simulink model "c_citation"  (R2020a)
settings: Solver=ode5  StartTime=0.0  StopTime=inf  FixedStep=0.01  RelTol=1e-3
InitFcn:
  | load('simulation_parameters');
values from neighbouring files (symbols this model uses):
  chord = 1.991    [citdata.mat]
  cv1 = 20000    [gear_params.m]
  cv2 = cv1    (= 20000)    [gear_params.m]
  cv3 = 4000    [gear_params.m]
  cv4 = 20000    [gear_params.m]
  deltagmax1 = 0.25    [gear_params.m]
  deltagmax2 = deltagmax1    (= 0.25)    [gear_params.m]
  deltagmax3 = 0.24    [gear_params.m]
  deltagmax4 = 0.02    [gear_params.m]
  ealphag = [0  0.2618  0.6981; 1  1.3  0.8]    [citdata.mat]
  ealphas = [0  0.2618  0.6981; 0.157  0.157  0.175]    [citdata.mat]
  g0 = 9.80665    [ac_genrl.mat]
  hDME = 0    [ac_genrl.mat]
  hGS = 0    [ac_genrl.mat]
  kt1 = 525020    [gear_params.m]
  kt2 = kt1    (= 525020)    [gear_params.m]
  kt3 = 457050    [gear_params.m]
  lh = 5.53    [citdata.mat]
  matbuaf = [0  -0.1745  0.4363; 0  -0.1  -0.1; 0.6981  -0.1  -0.1]    [citdata.mat]
  matdaf = [0 0 0.2618 0.6981 0.734842105263 0.771584210526 0.808326315789 0.845068421053 0.881810526316 0.918552631579 0.955294736842 0.992036842105 ... (529 elements, 23x23)]    [citdata.mat]
  matdam = [0 0.05 0.15 0.25 0.35 0.45 0.55 0.65 0.75 0.803571428571 0.857142857143 0.910714285714 ... (529 elements, 23x23)]    [citdata.mat]
  matdbbf = [0 0 0.6981 0.74464 0.79118 0.83772 0.88426 0.9308 0.97734 1.02388 1.07042 1.11696 ... (324 elements, 18x18)]    [citdata.mat]
  matdeaf = [0 0 0.2618 0.6981 0.734842105263 0.771584210526 0.808326315789 0.845068421053 0.881810526316 0.918552631579 0.955294736842 0.992036842105 ... (529 elements, 23x23)]    [citdata.mat]
  matdgaf = [0 0 0.2618 0.6981 -0.1745 -0.0175 -0.008 -0.009 0.4363 -0.0175 -0.008 -0.009 ... (16 elements, 4x4)]    [citdata.mat]
  matdqaf = [0 0 0.2618 0.6981 0.734842105263 0.771584210526 0.808326315789 0.845068421053 0.881810526316 0.918552631579 0.955294736842 0.992036842105 ... (529 elements, 23x23)]    [citdata.mat]
  matduaf = [0 0 0.2618 0.6981 0.734842105263 0.771584210526 0.808326315789 0.845068421053 0.881810526316 0.918552631579 0.955294736842 0.992036842105 ... (529 elements, 23x23)]    [citdata.mat]
  matdwaw = [0 0 0.1745 0.3491 0.5236 0.6458 1.2916 -0.1745 0 0.0018 0.0046 0.0088 ... (49 elements, 7x7)]    [citdata.mat]
  matedhr = [0 1 1 0.71 2 0.51 3 0.34 5 0.12 7.5 0.03 ... (20 elements, 2x10)]    [citdata.mat]
  mateif = [0  0.2618  0.6981; 0  -0.075  -0.075]    [citdata.mat]
  matelhr = [0 1 1 0.95 2 0.91 3 0.84 5 0.71 7.5 0.35 ... (20 elements, 2x10)]    [citdata.mat]
  matemhr = [0 1 1 0.9 2 0.8 3 0.7 5 0.5 7.5 0.25 ... (20 elements, 2x10)]    [citdata.mat]
  matemv1 = [0  90  100; 0  1  1]    [citdata.mat]
  matemv2 = [20  75  90; 0  1  1]    [citdata.mat]
  matemve = [0  90  100; 0  1  1]    [citdata.mat]
  matetam = [0  -0.1745  0.4363; 0  -0.04  -0.04; 1  -0.04  -0.04]    [citdata.mat]
  mateuaf = [0 0 0.6981 0.733005 0.76791 0.802815 0.83772 0.872625 0.90753 0.942435 0.97734 1.012245 ... (529 elements, 23x23)]    [citdata.mat]
  matfaaf = [0 0 0.2618 0.6981 0.734842105263 0.771584210526 0.808326315789 0.845068421053 0.881810526316 0.918552631579 0.955294736842 0.992036842105 ... (529 elements, 23x23)]    [citdata.mat]
  matfaxl = [0.15  0.35; 1  1]    [citdata.mat]
  matibaf = [0 0 0.2618 0.6981 -0.2 -0.119 -0.117 -0.108 0.3 -0.059 -0.052 -0.038 ... (16 elements, 4x4)]    [citdata.mat]
  matibb = [0 0 0.2618 1.571 3.142 -0.2 0 0 0.074 0.124 0 0 ... (50 elements, 5x10)]    [citdata.mat]
  matibmh = [0 0 15000 17142.8571429 19285.7142857 21428.5714286 23571.4285714 25714.2857143 27857.1428571 30000 0 0 ... (100 elements, 10x10)]    [citdata.mat]
  matipaf = [0  -0.1745  0.4363; 0  -0.44  -0.44; 0.6981  -0.44  -0.44]    [citdata.mat]
  matipmh = [0 0 15000 17142.8571429 19285.7142857 21428.5714286 23571.4285714 25714.2857143 27857.1428571 30000 0 0 ... (100 elements, 10x10)]    [citdata.mat]
  matiraf = [0 0 0.2618 0.6981 -0.2 0.05 -0.03 0.01 0.3 0.3 0.37 0.41 ... (16 elements, 4x4)]    [citdata.mat]
  matiuaf = [0  -0.2  0.3; 0  0.052  -0.003; 0.6981  0.052  -0.003]    [citdata.mat]
  matiwaf = [0  -0.1745  0.4363; 0  -0.185  -0.185; 0.6981  -0.185  -0.185]    [citdata.mat]
  matlaf = [0 0 0.2618 0.6981 0.734842105263 0.771584210526 0.808326315789 0.845068421053 0.881810526316 0.918552631579 0.955294736842 0.992036842105 ... (529 elements, 23x23)]    [citdata.mat]
  matlam = [0 0.05 0.15 0.25 0.35 0.45 0.55 0.65 0.75 0.803571428571 0.857142857143 0.910714285714 ... (529 elements, 23x23)]    [citdata.mat]
  matleaf = [0 0 0.2618 0.6981 0.734842105263 0.771584210526 0.808326315789 0.845068421053 0.881810526316 0.918552631579 0.955294736842 0.992036842105 ... (529 elements, 23x23)]    [citdata.mat]
  matleam = [0  -0.1745  0.4363; 0  0.58  0.58; 1  0.58  0.58]    [citdata.mat]
  matlgaf = [0 0 0.2618 0.6981 -0.1745 0.045 0.105 0.14 0.4363 0.045 0.105 0.14 ... (16 elements, 4x4)]    [citdata.mat]
  matlqaf = [0 0 0.2618 0.6981 0.734842105263 0.771584210526 0.808326315789 0.845068421053 0.881810526316 0.918552631579 0.955294736842 0.992036842105 ... (529 elements, 23x23)]    [citdata.mat]
  matluaf = [0 0 0.2618 0.6981 0.734842105263 0.771584210526 0.808326315789 0.845068421053 0.881810526316 0.918552631579 0.955294736842 0.992036842105 ... (529 elements, 23x23)]    [citdata.mat]
  matmaaf = [0 0 0.2618 0.6981 0.734842105263 0.771584210526 0.808326315789 0.845068421053 0.881810526316 0.918552631579 0.955294736842 0.992036842105 ... (484 elements, 22x22)]    [citdata.mat]
  matmaam = [0 0.05 0.15 0.25 0.35 0.45 0.55 0.65 0.75 0.803571428571 0.857142857143 0.910714285714 ... (484 elements, 22x22)]    [citdata.mat]
  matmaf = [0 0 0.2618 0.6981 0.734842105263 0.771584210526 0.808326315789 0.845068421053 0.881810526316 0.918552631579 0.955294736842 0.992036842105 ... (529 elements, 23x23)]    [citdata.mat]
  matmam = [0 0.05 0.15 0.25 0.35 0.45 0.55 0.65 0.75 0.803571428571 0.857142857143 0.910714285714 ... (529 elements, 23x23)]    [citdata.mat]
  matmbbf = [0 0 0.6981 0.74464 0.79118 0.83772 0.88426 0.9308 0.97734 1.02388 1.07042 1.11696 ... (324 elements, 18x18)]    [citdata.mat]
  matmeaf = [0 0 0.2618 0.6981 0.734842105263 0.771584210526 0.808326315789 0.845068421053 0.881810526316 0.918552631579 0.955294736842 0.992036842105 ... (529 elements, 23x23)]    [citdata.mat]
  matmeam = [0 0 1 1.05 1.1 1.15 1.2 1.25 1.3 1.35 1.4 1.45 ... (529 elements, 23x23)]    [citdata.mat]
  matmgaf = [0 0 0.2618 0.6981 -0.1745 -0.01 -0.024 -0.035 0.4363 -0.01 -0.024 -0.035 ... (16 elements, 4x4)]    [citdata.mat]
  matmqaf = [0 0 0.2618 0.6981 0.734842105263 0.771584210526 0.808326315789 0.845068421053 0.881810526316 0.918552631579 0.955294736842 0.992036842105 ... (529 elements, 23x23)]    [citdata.mat]
  matmrbr = [0  0  0.5236; 0  0  0; 0.384  0.001  0.001]    [citdata.mat]
  matnbab = [0 0 0.2618 1.571 3.142 -0.2 0 0 -0.0199 -0.1049 0 0 ... (25 elements, 5x5)]    [citdata.mat]
  matnbaf = [0  -0.2  0.3; 0  0.105  0.18; 0.6981  0.105  0.18]    [citdata.mat]
  matnbmh = [0 0 15000 17142.8571429 19285.7142857 21428.5714286 23571.4285714 25714.2857143 27857.1428571 30000 0 0 ... (100 elements, 10x10)]    [citdata.mat]
  matnpaf = [0 0 0.2618 0.6981 -0.2 0.03 0.03 0.05 0.3 -0.12 -0.12 -0.2 ... (16 elements, 4x4)]    [citdata.mat]
  matnpmh = [0 0 15000 17142.8571429 19285.7142857 21428.5714286 23571.4285714 25714.2857143 27857.1428571 30000 0 0 ... (100 elements, 10x10)]    [citdata.mat]
  matnraf = [0  -0.1745  0.4363; 0  -0.21  -0.21; 0.6981  -0.21  -0.21]    [citdata.mat]
  matnuaf = [0  -0.1745  0.4363; 0  -0.101  -0.101; 0.6981  -0.101  -0.101]    [citdata.mat]
  matnwaf = [0 0 0.2618 0.6981 -0.2 -0.02 -0.037 -0.049 0.3 0.03 0.043 0.036 ... (16 elements, 4x4)]    [citdata.mat]
  matnwmh = [0 0 15000 17142.8571429 19285.7142857 21428.5714286 23571.4285714 25714.2857143 27857.1428571 30000 0 0 ... (100 elements, 10x10)]    [citdata.mat]
  matqlaf = [0  -0.1745  0.4363; 0  -1  -1; 0.6981  -1  -1]    [citdata.mat]
  matquaf = [0 0 0.6981 0.733005 0.76791 0.802815 0.83772 0.872625 0.90753 0.942435 0.97734 1.012245 ... (529 elements, 23x23)]    [citdata.mat]
  matqxl = [0.15  0.35; 1  1]    [citdata.mat]
  matqxm = [0.15  0.35; 1  1]    [citdata.mat]
  matrtam = [0  -0.1745  0.4363; 0  0.011  0.011; 1  0.011  0.011]    [citdata.mat]
  matruaf = [0  -0.1745  0.4363; 0  0.2  0.2; 0.6981  0.2  0.2]    [citdata.mat]
  matrumh = [0 0 15000 17142.8571429 19285.7142857 21428.5714286 23571.4285714 25714.2857143 27857.1428571 30000 0 0 ... (100 elements, 10x10)]    [citdata.mat]
  matuut = [0  0.5  1; 0  1.35  1]    [citdata.mat]
  matwtam = [0  -0.1745  0.4363; 0  0.011  0.011; 1  0.011  0.011]    [citdata.mat]
  matybab = [0 0 0.2618 1.571 3.142 -0.2 0 0 0.34 0.75 0 0 ... (25 elements, 5x5)]    [citdata.mat]
  matybaf = [0  -0.1745  0.4363; 0  -0.75  -0.75; 0.6981  -0.75  -0.75]    [citdata.mat]
  matyraf = [0  -0.1745  0.4363; 0  0.85  0.85; 0.6981  0.85  0.85]    [citdata.mat]
  matyuaf = [0  -0.1745  0.4363; 0  0.23  0.23; 0.6981  0.23  0.23]    [citdata.mat]
  matywaf = [0  -0.1745  0.4363; 0  -0.04  -0.04; 0.6981  -0.04  -0.04]    [citdata.mat]
  murol = 0.03*10    (= 0.3)    [gear_params.m]
  P1 = 2000    [gear_params.m]
  P2 = P1    (= 2000)    [gear_params.m]
  P3 = 2550    [gear_params.m]
  P4 = 40000    [gear_params.m]
  psiLOC = 0    [ac_genrl.mat]
  pstat0 = 101325    [ac_genrl.mat]
  S = 24.99    [citdata.mat]
  span = 13.325    [citdata.mat]
  T0 = 288.15    [ac_genrl.mat]
  tilteng = [0 0]    [citdata.mat]
  toweng = [0 0]    [citdata.mat]
  vdommyr37 = [0  0.2618  0.6981; 0  0.025  0]    [citdata.mat]
  vdommyr38 = [0  0.2618  0.6981; -0.01  0  -0.01]    [citdata.mat]
  Vw915 = 0    [initcit.m]
  winddir = 45*(pi/180)    (= 0.785398163397)    [initcit.m]
  xcgref = 6.5    [citdata.mat]
  xDME = 0    [ac_genrl.mat]
  xeng = [8.407 8.407]    [citdata.mat]
  xGS = 0    [ac_genrl.mat]
  xiacc = 3.2    [ac_genrl.mat]
  xl1 = xcg-6.858    [gear_params.m]
  xl2 = xcg-6.858    [gear_params.m]
  xl3 = xcg-2.0752    [gear_params.m]
  xl4 = xcg-12.742    [gear_params.m]
  xLOC = 0    [ac_genrl.mat]
  ycgref = 0    [citdata.mat]
  yDME = 0    [ac_genrl.mat]
  yeng = [3 -3]    [citdata.mat]
  yGS = 0    [ac_genrl.mat]
  yiacc = 0    [ac_genrl.mat]
  yl1 = 1.918    [gear_params.m]
  yl2 = -1.918    [gear_params.m]
  yl3 = 0    [gear_params.m]
  ... (+9 more)
undefined symbols (not defined in the file or in its folder): Deng, massinit, matff, matn1d, matn2d, matthr, u0, ut0, x0, xt0
(part 3 of 5)

== system c_citation/Cessna Citation 500/Citation model DASMAT/AIRCRAFT MODEL/LANDING GEAR/Landing Gear model/Left Main Gear ==
  Inputs : Inport
  Axes Transformation Heading attached vertical axis to body axis : Subsystem
  Calculation of the Moments : Subsystem
  Demux : Demux  Outputs=[6 2 5]
      settings: DisplayOption=none
  FS Side Force : Constant  Value=0
  FV Vertical Force : Subsystem
  Fmu Longitudinal Force : Fcn  Expr=u[1]*murol
  Mux : Mux  Inputs=3
  Mux1 : Mux  Inputs=2
  Terminator : Terminator
  Terminator1 : Terminator
  FX FY FZ : Outport  VectorParamsAs1DForOutWhenUnconnected=off
  L M N : Outport  Port=2  VectorParamsAs1DForOutWhenUnconnected=off
  wires:
  Fmu Longitudinal Force/1 -> Mux/1
  FS Side Force/1 -> Mux/2
  FV Vertical Force/1(Out1) -> Fmu Longitudinal Force/1, Mux/3
  Calculation of the Moments/1(L M N) -> L M N/1
  Inputs/1 -> FV Vertical Force/1(In1), Demux/1
  Demux/1 -> Terminator/1
  Demux/3 -> Terminator1/1
  Mux1/1 -> Axes Transformation Heading attached vertical axis to body axis/1(Fmu FS FV phi theta)
  Mux/1 -> Mux1/1
  Demux/2 -> Mux1/2  "phi theta"
  Axes Transformation Heading attached vertical axis to body axis/1(FX FY FZ) -> FX FY FZ/1, Calculation of the Moments/1(FX FY FZ)

== system c_citation/Cessna Citation 500/Citation model DASMAT/AIRCRAFT MODEL/LANDING GEAR/Landing Gear model/Nose Gear ==
  Inputs : Inport
  Axes Transformation Heading attached vertical axis to body axis : Subsystem
  Calculation of the Moments : Subsystem
  Demux : Demux  Outputs=[6 2 5]
      settings: DisplayOption=none
  F Vertical Force : Subsystem
  FS Side Force : Constant  Value=0
  Fmu Longitudinal Force : Fcn  Expr=u[1]*murol
  Mux : Mux  Inputs=3
  Mux1 : Mux  Inputs=2
  Terminator : Terminator
  Terminator1 : Terminator
  FX FY FZ : Outport  VectorParamsAs1DForOutWhenUnconnected=off
  L M N : Outport  Port=2  VectorParamsAs1DForOutWhenUnconnected=off
  wires:
  Fmu Longitudinal Force/1 -> Mux/1
  FS Side Force/1 -> Mux/2
  F Vertical Force/1(Out1) -> Fmu Longitudinal Force/1, Mux/3
  Calculation of the Moments/1(L M N) -> L M N/1
  Inputs/1 -> F Vertical Force/1(In1), Demux/1
  Demux/1 -> Terminator/1
  Demux/3 -> Terminator1/1
  Mux1/1 -> Axes Transformation Heading attached vertical axis to body axis/1(Fmu FS FV phi theta)
  Mux/1 -> Mux1/1
  Demux/2 -> Mux1/2  "phi theta"
  Axes Transformation Heading attached vertical axis to body axis/1(FX FY FZ) -> FX FY FZ/1, Calculation of the Moments/1(FX FY FZ)

== system c_citation/Cessna Citation 500/Citation model DASMAT/AIRCRAFT MODEL/LANDING GEAR/Landing Gear model/Right Main Gear ==
  Inputs : Inport
  Axes Transformation Heading attached vertical axis to body axis : Subsystem
  Calculation of the Moments : Subsystem
  Demux : Demux  Outputs=[6 2 5]
      settings: DisplayOption=none
  FS Side Force : Constant  Value=0
  FV Vertical Force : Subsystem
  Fmu Longitudinal Force : Fcn  Expr=u[1]*murol
  Mux : Mux  Inputs=3
  Mux1 : Mux  Inputs=2
  Terminator : Terminator
  Terminator1 : Terminator
  FX FY FZ : Outport  VectorParamsAs1DForOutWhenUnconnected=off
  L M N : Outport  Port=2  VectorParamsAs1DForOutWhenUnconnected=off
  wires:
  Fmu Longitudinal Force/1 -> Mux/1
  FS Side Force/1 -> Mux/2
  FV Vertical Force/1(Out1) -> Fmu Longitudinal Force/1, Mux/3
  Calculation of the Moments/1(L M N) -> L M N/1
  Inputs/1 -> FV Vertical Force/1(In1), Demux/1
  Demux/1 -> Terminator/1
  Demux/3 -> Terminator1/1
  Mux1/1 -> Axes Transformation Heading attached vertical axis to body axis/1(Fmu FS FV phi theta)
  Mux/1 -> Mux1/1
  Demux/2 -> Mux1/2  "phi theta"
  Axes Transformation Heading attached vertical axis to body axis/1(FX FY FZ) -> FX FY FZ/1, Calculation of the Moments/1(FX FY FZ)

== system c_citation/Cessna Citation 500/Citation model DASMAT/AIRCRAFT MODEL/LANDING GEAR/Landing Gear model/Tail Scraper ==
  Inputs : Inport
  Axes Transformation Heading attached vertical axis to body axis : Subsystem
  Calculation of the Moments : Subsystem
  Demux : Demux  Outputs=[6 2 5]
      settings: DisplayOption=none
  FS Side Force : Constant  Value=0
  FV Vertical Force : Subsystem
  Fmu : Constant  Value=0
  Mux : Mux  Inputs=3
  Mux1 : Mux  Inputs=2
  Terminator : Terminator
  Terminator1 : Terminator
  FX FY FZ : Outport  VectorParamsAs1DForOutWhenUnconnected=off
  L M N : Outport  Port=2  VectorParamsAs1DForOutWhenUnconnected=off
  wires:
  Fmu/1 -> Mux/1
  FS Side Force/1 -> Mux/2
  Calculation of the Moments/1(L M N) -> L M N/1
  Inputs/1 -> FV Vertical Force/1(In1), Demux/1
  Demux/1 -> Terminator/1
  Demux/3 -> Terminator1/1
  Mux1/1 -> Axes Transformation Heading attached vertical axis to body axis/1(Fmu FS FV phi theta)
  Mux/1 -> Mux1/1
  Demux/2 -> Mux1/2  "phi theta"
  Axes Transformation Heading attached vertical axis to body axis/1(FX FY FZ) -> FX FY FZ/1, Calculation of the Moments/1(FX FY FZ)
  FV Vertical Force/1(Out1) -> Mux/3

== system c_citation/Cessna Citation 500/Citation model DASMAT/AIRCRAFT MODEL/WIND//TURBULENCE/Logarithmic Wind model/Logarithmic Wind model ==
  note: winddir output deleted
      | you can calculate it yourself
      | from uvw, you lazy bastard
  note: runway elevation
      | correction deleted,
      | is all relative to sea level
  he : Inport
  Constant : Constant  Value=0
  Mux : Mux  Inputs=2
  Product : Product  InputSameDT=on  SaturateOnIntegerOverflow=on  OutDataTypeStr=Inherit: Same as first input
  Switch : Switch  Threshold=300  SaturateOnIntegerOverflow=on  InputSameDT=on
  Vwind above 300m : Fcn  Expr=1.637
  Vwind below 300m : Fcn  Expr=(0.43*log10(u)+0.572)
  Vwind915 : Subsystem
  Windddirection : Subsystem
  uwind earth axis : Fcn  Expr=cos(u[1])*u[2]
  vwind earth axis : Fcn  Expr=sin(u[1])*u[2]
  uwind : Outport  VectorParamsAs1DForOutWhenUnconnected=off
  vwind : Outport  Port=2  VectorParamsAs1DForOutWhenUnconnected=off
  wwind : Outport  Port=3  VectorParamsAs1DForOutWhenUnconnected=off
  wires:
  Vwind above 300m/1 -> Switch/1
  Vwind below 300m/1 -> Switch/3
  Constant/1 -> wwind/1
  he/1 -> Switch/2, Vwind above 300m/1, Vwind below 300m/1
  Switch/1 -> Product/2
  Vwind915/1(Out1) -> Product/1
  Product/1 -> Mux/2
  Windddirection/1(Out1) -> Mux/1
  uwind earth axis/1 -> uwind/1
  vwind earth axis/1 -> vwind/1
  Mux/1 -> uwind earth axis/1, vwind earth axis/1

== system c_citation/Cessna Citation 500/Citation model DASMAT/AIRCRAFT MODEL/AFM/Aeromod/SubSystem/Ground effect ==
  yatm : Inport
  Sat : Saturate  UpperLimit=21  LowerLimit=-inf
  radio alt selector : Selector  IndexOptions=Index vector (dialog)  Indices=[6]  OutputSizes=1
  hcg : Outport  VectorParamsAs1DForOutWhenUnconnected=off
  wires:
  radio alt selector/1 -> Sat/1
  Sat/1 -> hcg/1
  yatm/1 -> radio alt selector/1

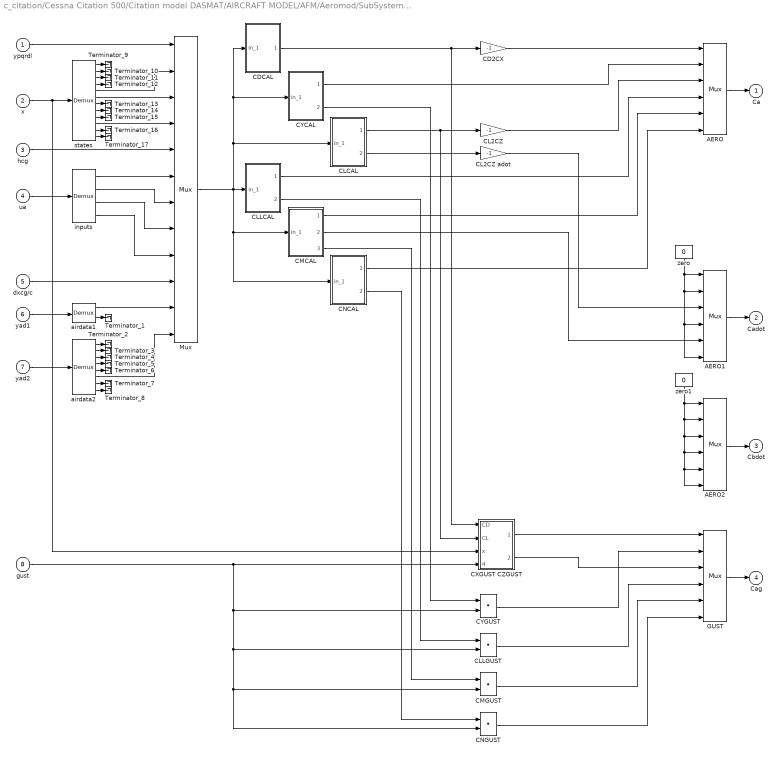
== system c_citation/Cessna Citation 500/Citation model DASMAT/AIRCRAFT MODEL/AFM/Aeromod/SubSystem/model ==
  ypqrdl : Inport
  x : Inport  Port=2
  hcg : Inport  Port=3
  ua : Inport  Port=4
  dxcg/c : Inport  Port=5
  yad1 : Inport  Port=6
  yad2 : Inport  Port=7
  gust : Inport  Port=8
  AERO : Mux  Inputs=6
  AERO1 : Mux  Inputs=6
  AERO2 : Mux  Inputs=6
  CD2CX : Gain  Gain=-1  SaturateOnIntegerOverflow=on  OutDataTypeStr=Inherit: Same as input  ParamDataTypeStr=Inherit: Same as input
  CDCAL : Subsystem
  CL2CZ : Gain  Gain=-1  SaturateOnIntegerOverflow=on  OutDataTypeStr=Inherit: Same as input  ParamDataTypeStr=Inherit: Same as input
  CL2CZ adot : Gain  Gain=-1  SaturateOnIntegerOverflow=on  OutDataTypeStr=Inherit: Same as input  ParamDataTypeStr=Inherit: Same as input
  CLCAL : Subsystem
  CLLCAL : Subsystem
  CLLGUST : DotProduct  InputSameDT=on  OutDataTypeStr=Inherit: Inherit via internal rule
  CMCAL : Subsystem
  CMGUST : DotProduct  InputSameDT=on  OutDataTypeStr=Inherit: Inherit via internal rule
  CNCAL : Subsystem
  CNGUST : DotProduct  InputSameDT=on  OutDataTypeStr=Inherit: Inherit via internal rule
  CXGUST CZGUST : Subsystem
  CYCAL : Subsystem
  CYGUST : DotProduct  InputSameDT=on  OutDataTypeStr=Inherit: Inherit via internal rule
  GUST : Mux  Inputs=6
  Mux : Mux  Inputs=[3 1 1 1 1 3 3 1 1 1 1 1]
  Terminator_{1..17} (17 alike) : Terminator
  airdata1 : Demux  Outputs=2
      settings: DisplayOption=none
  airdata2 : Demux  Outputs=8
      settings: DisplayOption=none
  inputs : Demux  Outputs=[3 3 1 1]
      settings: DisplayOption=none
  states : Demux  Outputs=12
      settings: DisplayOption=none
  zero : Constant  Value=0
  zero1 : Constant  Value=0
  Ca : Outport  VectorParamsAs1DForOutWhenUnconnected=off
  Cadot : Outport  Port=2  VectorParamsAs1DForOutWhenUnconnected=off
  Cbdot : Outport  Port=3  VectorParamsAs1DForOutWhenUnconnected=off
  Cag : Outport  Port=4  VectorParamsAs1DForOutWhenUnconnected=off
  wires:
  states/12 -> Terminator_17/1
  states/11 -> Terminator_16/1
  states/9 -> Terminator_15/1
  states/8 -> Terminator_14/1
  states/7 -> Terminator_13/1
  states/4 -> Terminator_12/1
  states/3 -> Terminator_11/1
  states/2 -> Terminator_10/1
  states/1 -> Terminator_9/1
  airdata2/8 -> Terminator_8/1
  airdata2/7 -> Terminator_7/1
  airdata2/5 -> Terminator_6/1
  airdata2/4 -> Terminator_5/1
  airdata2/3 -> Terminator_4/1
  airdata2/2 -> Terminator_3/1
  airdata2/1 -> Terminator_2/1
  airdata1/2 -> Terminator_1/1
  gust/1 -> CYGUST/2, CLLGUST/2, CMGUST/2, CNGUST/2, CXGUST CZGUST/4(gust)
  x/1 -> CXGUST CZGUST/3(x), states/1
  airdata1/1 -> Mux/11
  CDCAL/1(out_1) -> CXGUST CZGUST/1(CD), CD2CX/1
  CNCAL/2("out_2 ") -> CNGUST/1
  CMCAL/3("out_3 ") -> CMGUST/1
  CMCAL/2(out_2) -> AERO1/5
  CMCAL/1(out_1) -> AERO/5
  CNCAL/1(out_1) -> AERO/6
  CLLCAL/2(out_2) -> CLLGUST/1
  CLLCAL/1(out_1) -> AERO/4
  CLCAL/2(out_2) -> CL2CZ adot/1
  CYCAL/2(out_2) -> CYGUST/1
  CYCAL/1(out_1) -> AERO/2
  CL2CZ adot/1 -> AERO1/3
  CNGUST/1 -> GUST/6
  CLLGUST/1 -> GUST/4
  CMGUST/1 -> GUST/5
  CYGUST/1 -> GUST/2
  CLCAL/1(out_1) -> CXGUST CZGUST/2(CL), CL2CZ/1
  CL2CZ/1 -> AERO/3
  CD2CX/1 -> AERO/1
  airdata2/6 -> Mux/12
  CXGUST CZGUST/2("out_2 ") -> GUST/3
  GUST/1 -> Cag/1
  AERO/1 -> Ca/1
  Mux/1 -> CMCAL/1(in_1), CNCAL/1(in_1), CLCAL/1(in_1), CYCAL/1(in_1), CDCAL/1(in_1), CLLCAL/1(in_1)
  CXGUST CZGUST/1("out_1 ") -> GUST/1
  yad2/1 -> airdata2/1
  inputs/3 -> Mux/8
  hcg/1 -> Mux/5
  ua/1 -> inputs/1
  yad1/1 -> airdata1/1
  dxcg/c/1 -> Mux/10
  states/6 -> Mux/3
  states/10 -> Mux/4
  ypqrdl/1 -> Mux/1
  inputs/1 -> Mux/6
  states/5 -> Mux/2
  inputs/4 -> Mux/9
  inputs/2 -> Mux/7
  AERO1/1 -> Cadot/1
  zero/1 -> AERO1/4, AERO1/6, AERO1/2, AERO1/1
  zero1/1 -> AERO2/1, AERO2/2, AERO2/3, AERO2/4, AERO2/5, AERO2/6
  AERO2/1 -> Cbdot/1

== system c_citation/Cessna Citation 500/Citation model DASMAT/AIRCRAFT MODEL/AFM/Aeromod/SubSystem/pqrnondims ==
  x : Inport
  Demux : Demux  Outputs=[3 3 3 3]
      settings: DisplayOption=none
  Mux : Mux  Inputs=[12 1 1 1]
  Mux1 : Mux  Inputs=3
  Prod : Product  InputSameDT=on  SaturateOnIntegerOverflow=on  OutDataTypeStr=Inherit: Same as first input
  Terminator_{1..12} (12 alike) : Terminator
  b/2V : Fcn  Expr=span/(2*u[4])
  b/2V1 : Fcn  Expr=span/(2*u[4])
  c/V : Fcn  Expr=chord/u[4]
  pqr transformation : S-Function  FunctionName=ac_axes  Parameters=2  SFunctionDeploymentMode=off  EnableBusSupport=off
  states : Demux  Outputs=12
      settings: DisplayOption=none
  ypqrdl : Outport  VectorParamsAs1DForOutWhenUnconnected=off
  wires:
  states/12 -> Terminator_12/1
  states/11 -> Terminator_11/1
  states/10 -> Terminator_10/1
  states/9 -> Terminator_9/1
  states/8 -> Terminator_8/1
  states/7 -> Terminator_7/1
  states/6 -> Terminator_6/1
  states/5 -> Terminator_5/1
  states/4 -> Terminator_4/1
  Demux/4 -> Terminator_3/1
  Demux/3 -> Terminator_2/1
  Demux/1 -> Terminator_1/1
  Mux/1 -> pqr transformation/1
  states/1 -> Mux/2
  states/2 -> Mux/3
  states/3 -> Mux/4
  Prod/1 -> ypqrdl/1
  Mux1/1 -> Prod/2
  x/1 -> states/1, b/2V/1, b/2V1/1, c/V/1, Mux/1
  b/2V/1 -> Mux1/1
  b/2V1/1 -> Mux1/3
  c/V/1 -> Mux1/2
  pqr transformation/1 -> Demux/1
  Demux/2 -> Prod/1

== system c_citation/Cessna Citation 500/Citation model DASMAT/AIRCRAFT MODEL/AFM/Aeromod/SubSystem/rud-rudtrim coupling ==
  ua : Inport
  Demux : Demux  Outputs=[3 1 1 1 2]
      settings: DisplayOption=none
  Mux : Mux  Inputs=[3 1 1 1 2]
  Terminator_1 : Terminator
  rud-rudtrim coupled : Fcn  Expr=u[6]+0.536*u[3]
  ua coupled : Outport  VectorParamsAs1DForOutWhenUnconnected=off
  wires:
  Demux/4 -> Terminator_1/1
  Mux/1 -> ua coupled/1
  Demux/5 -> Mux/5
  Demux/3 -> Mux/3
  Demux/2 -> Mux/2
  rud-rudtrim coupled/1 -> Mux/4
  Demux/1 -> Mux/1
  ua/1 -> rud-rudtrim coupled/1, Demux/1

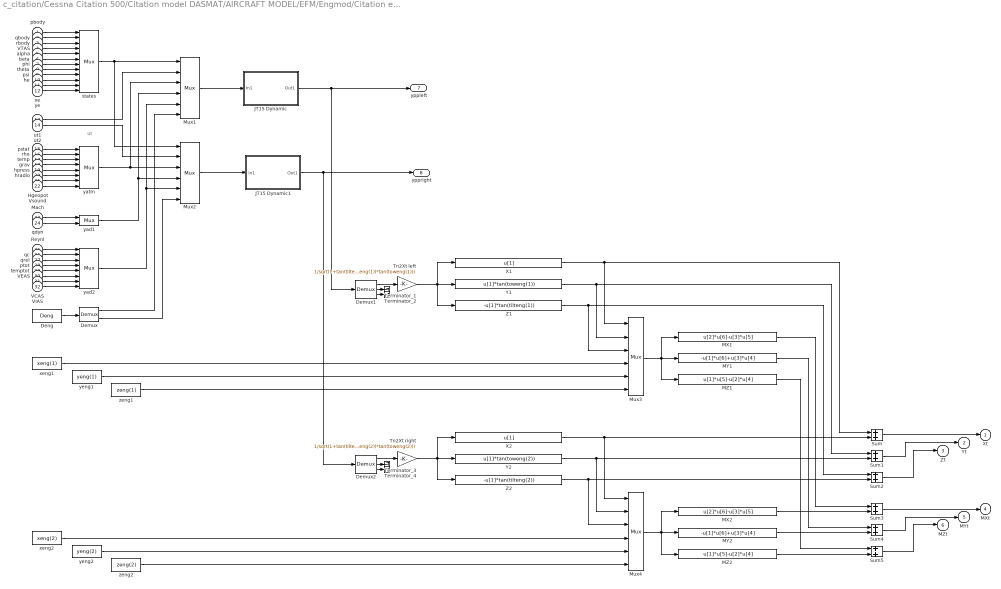
== system c_citation/Cessna Citation 500/Citation model DASMAT/AIRCRAFT MODEL/EFM/Engmod/Citation eng_mod/Subsystem1 ==
  note: ut
  pbody : Inport
  qbody : Inport  Port=2
  rbody : Inport  Port=3
  VTAS : Inport  Port=4
  alpha : Inport  Port=5
  beta : Inport  Port=6
  phi : Inport  Port=7
  theta : Inport  Port=8
  psi : Inport  Port=9
  he : Inport  Port=10
  xe : Inport  Port=11
  ye : Inport  Port=12
  ut1 : Inport  Port=13
  ut2 : Inport  Port=14
  pstat : Inport  Port=15
  rho : Inport  Port=16
  temp : Inport  Port=17
  grav : Inport  Port=18
  hpress : Inport  Port=19
  hradio : Inport  Port=20
  Hgeopot : Inport  Port=21
  Vsound : Inport  Port=22
  Mach : Inport  Port=23
  qdyn : Inport  Port=24
  Reynl : Inport  Port=25
  qc : Inport  Port=26
  qrel : Inport  Port=27
  ptot : Inport  Port=28
  temptot : Inport  Port=29
  VEAS : Inport  Port=30
  VCAS : Inport  Port=31
  VIAS : Inport  Port=32
  Demux : Demux  Outputs=2
      settings: DisplayOption=none
  Demux1 : Demux  Outputs=[1 1 -1]
      settings: DisplayOption=none
  Demux2 : Demux  Outputs=[1 1 -1]
      settings: DisplayOption=none
  Deng : Constant  Value=Deng
  JT15 Dynamic : Subsystem
  JT15 Dynamic1 : Subsystem
  MX1 : Fcn  Expr=u[2]*u[6]-u[3]*u[5]
  MX2 : Fcn  Expr=u[2]*u[6]-u[3]*u[5]
  MY1 : Fcn  Expr=-u[1]*u[6]+u[3]*u[4]
  MY2 : Fcn  Expr=-u[1]*u[6]+u[3]*u[4]
  MZ1 : Fcn  Expr=u[1]*u[5]-u[2]*u[4]
  MZ2 : Fcn  Expr=u[1]*u[5]-u[2]*u[4]
  Mux1 : Mux  Inputs=[12 1 8 2 8 1]
  Mux2 : Mux  Inputs=[12 1 8 2 8 1]
  Mux3 : Mux  Inputs=6
  Mux4 : Mux  Inputs=6
  Sum{,1..5} (6 alike) : Sum  InputSameDT=on  SaturateOnIntegerOverflow=on  OutDataTypeStr=Inherit: Same as first input
  Terminator_{1..4} (4 alike) : Terminator
  Tn2Xt left : Gain  Gain=1/sqrt(1+tan(tilteng(1))*tan(tilteng(1))+tan(toweng(1))*tan(toweng(1)))  SaturateOnIntegerOverflow=on  OutDataTypeStr=Inherit: Same as input  ParamDataTypeStr=Inherit: Same as input
  Tn2Xt right : Gain  Gain=1/sqrt(1+tan(tilteng(2))*tan(tilteng(2))+tan(toweng(2))*tan(toweng(2)))  SaturateOnIntegerOverflow=on  OutDataTypeStr=Inherit: Same as input  ParamDataTypeStr=Inherit: Same as input
  X1 : Fcn  Expr=u[1]
  X2 : Fcn  Expr=u[1]
  Y1 : Fcn  Expr=u[1]*tan(toweng(1))
  Y2 : Fcn  Expr=u[1]*tan(toweng(2))
  Z1 : Fcn  Expr=-u[1]*tan(tilteng(1))
  Z2 : Fcn  Expr=-u[1]*tan(tilteng(2))
  states : Mux  Inputs=12
  xeng1 : Constant  Value=xeng(1)
  xeng2 : Constant  Value=xeng(2)
  yad1 : Mux  Inputs=2
  yad2 : Mux  Inputs=8
  yatm : Mux  Inputs=8
  yeng1 : Constant  Value=yeng(1)
  yeng2 : Constant  Value=yeng(2)
  zeng1 : Constant  Value=zeng(1)
  zeng2 : Constant  Value=zeng(2)
  Xt : Outport  VectorParamsAs1DForOutWhenUnconnected=off
  Yt : Outport  Port=2  VectorParamsAs1DForOutWhenUnconnected=off
  Zt : Outport  Port=3  VectorParamsAs1DForOutWhenUnconnected=off
  MXt : Outport  Port=4  VectorParamsAs1DForOutWhenUnconnected=off
  MYt : Outport  Port=5  VectorParamsAs1DForOutWhenUnconnected=off
  MZt : Outport  Port=6  VectorParamsAs1DForOutWhenUnconnected=off
  yppleft : Outport  Port=7  VectorParamsAs1DForOutWhenUnconnected=off
  yppright : Outport  Port=8  VectorParamsAs1DForOutWhenUnconnected=off
  wires:
  grav/1 -> yatm/4
  hradio/1 -> yatm/6
  temp/1 -> yatm/3
  hpress/1 -> yatm/5
  Hgeopot/1 -> yatm/7
  rho/1 -> yatm/2
  pstat/1 -> yatm/1
  pbody/1 -> states/1
  qbody/1 -> states/2
  phi/1 -> states/7
  alpha/1 -> states/5
  rbody/1 -> states/3
  theta/1 -> states/8
  beta/1 -> states/6
  VTAS/1 -> states/4
  psi/1 -> states/9
  he/1 -> states/10
  xe/1 -> states/11
  ye/1 -> states/12
  ptot/1 -> yad2/4
  VEAS/1 -> yad2/6
  VIAS/1 -> yad2/8
  qrel/1 -> yad2/3
  temptot/1 -> yad2/5
  VCAS/1 -> yad2/7
  qc/1 -> yad2/2
  Reynl/1 -> yad2/1
  qdyn/1 -> yad1/2
  Mux1/1 -> JT15 Dynamic/1(In1)
  Mux2/1 -> JT15 Dynamic1/1(In1)
  Tn2Xt left/1 -> Y1/1, X1/1, Z1/1
  xeng1/1 -> Mux3/4
  yeng1/1 -> Mux3/5
  zeng1/1 -> Mux3/6
  Mux3/1 -> MY1/1, MX1/1, MZ1/1
  zeng2/1 -> Mux4/6
  yeng2/1 -> Mux4/5
  xeng2/1 -> Mux4/4
  Tn2Xt right/1 -> Y2/1, Z2/1, X2/1
  MZ2/1 -> Sum5/2
  MY2/1 -> Sum4/2
  MX2/1 -> Sum3/2
  Mux4/1 -> MY2/1, MZ2/1, MX2/1
  MZ1/1 -> Sum5/1
  MY1/1 -> Sum4/1
  MX1/1 -> Sum3/1
  Y2/1 -> Sum1/2, Mux4/2
  X2/1 -> Sum/2, Mux4/1
  X1/1 -> Sum/1, Mux3/1
  Z1/1 -> Sum2/1, Mux3/3
  Y1/1 -> Sum1/1, Mux3/2
  Z2/1 -> Sum2/2, Mux4/3
  Sum/1 -> Xt/1
  Sum1/1 -> Yt/1
  Sum2/1 -> Zt/1
  Sum3/1 -> MXt/1
  Sum4/1 -> MYt/1
  Sum5/1 -> MZt/1
  ut1/1 -> Mux1/2
  yad1/1 -> Mux1/4, Mux2/4
  yad2/1 -> Mux1/5, Mux2/5
  yatm/1 -> Mux2/3, Mux1/3
  ut2/1 -> Mux2/2
  states/1 -> Mux1/1, Mux2/1
  Demux1/1 -> Tn2Xt left/1
  Demux2/1 -> Tn2Xt right/1
  Vsound/1 -> yatm/8
  Mach/1 -> yad1/1
  Deng/1 -> Demux/1
  Demux/1 -> Mux1/6
  Demux/2 -> Mux2/6
  Demux1/2 -> Terminator_1/1
  Demux1/3 -> Terminator_2/1
  Demux2/2 -> Terminator_3/1
  Demux2/3 -> Terminator_4/1
  JT15 Dynamic/1(Out1) -> Demux1/1, yppleft/1
  JT15 Dynamic1/1(Out1) -> Demux2/1, yppright/1

== system c_citation/Cessna Citation 500/Citation model DASMAT/AIRCRAFT MODEL/EQM/State Derivatives/Vabdot/Vdot ==
  x : Inport
  ypqr : Inport  Port=2
  Ftot : Inport  Port=3
  mass : Inport  Port=4
  wind : Inport  Port=5
  winddot : Inport  Port=6
  adot : Inport  Port=7
  bdot : Inport  Port=8
  Demux{,1..3} (4 alike) : Demux  Outputs=[3 3 3 3]
      settings: DisplayOption=none
  Mux2 : Mux  Inputs=[3 3 3 3 1 1 1 1 1]
  Terminator_{1..22} (22 alike) : Terminator
  VTASdot : Fcn  Expr=u[1]/u[17]-(u[10]+(u[5]-u[15]*cos(u[14]))*u[9]-(u[6]-u[16])*u[8])
  states : Demux  Outputs=12
      settings: DisplayOption=none
  Vdot : Outport  VectorParamsAs1DForOutWhenUnconnected=off
  wires:
  states/12 -> Terminator_22/1
  states/11 -> Terminator_21/1
  states/10 -> Terminator_20/1
  states/9 -> Terminator_19/1
  states/8 -> Terminator_18/1
  states/7 -> Terminator_17/1
  states/5 -> Terminator_16/1
  states/3 -> Terminator_15/1
  states/2 -> Terminator_14/1
  states/1 -> Terminator_13/1
  Demux3/4 -> Terminator_12/1
  Demux3/3 -> Terminator_11/1
  Demux3/2 -> Terminator_10/1
  Demux2/4 -> Terminator_9/1
  Demux2/3 -> Terminator_8/1
  Demux2/2 -> Terminator_7/1
  Demux1/4 -> Terminator_6/1
  Demux1/3 -> Terminator_5/1
  Demux1/2 -> Terminator_4/1
  Demux/4 -> Terminator_3/1
  Demux/3 -> Terminator_2/1
  Demux/2 -> Terminator_1/1
  Demux3/1 -> Mux2/4
  Mux2/1 -> VTASdot/1
  winddot/1 -> Demux3/1
  states/6 -> Mux2/6
  adot/1 -> Mux2/7
  mass/1 -> Mux2/9
  bdot/1 -> Mux2/8
  Demux2/1 -> Mux2/3
  states/4 -> Mux2/5
  wind/1 -> Demux2/1
  Ftot/1 -> Demux/1
  Demux/1 -> Mux2/1
  Demux1/1 -> Mux2/2
  ypqr/1 -> Demux1/1
  x/1 -> states/1
  VTASdot/1 -> Vdot/1

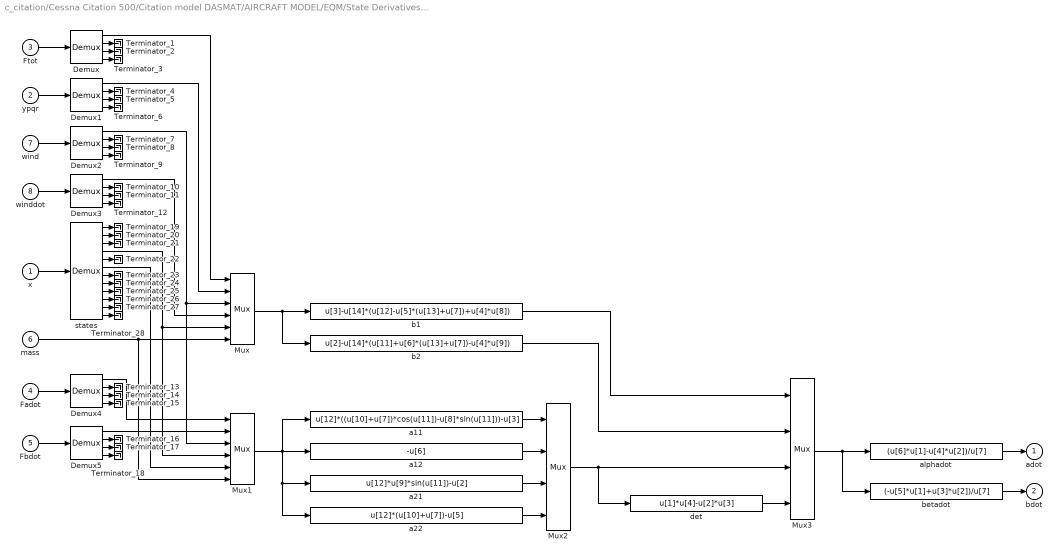
== system c_citation/Cessna Citation 500/Citation model DASMAT/AIRCRAFT MODEL/EQM/State Derivatives/Vabdot/abdot ==
  x : Inport
  ypqr : Inport  Port=2
  Ftot : Inport  Port=3
  Fadot : Inport  Port=4
  Fbdot : Inport  Port=5
  mass : Inport  Port=6
  wind : Inport  Port=7
  winddot : Inport  Port=8
  Demux{,1..5} (6 alike) : Demux  Outputs=[3 3 3 3]
      settings: DisplayOption=none
  Mux : Mux  Inputs=[3 3 3 3 1 1]
  Mux1 : Mux  Inputs=[3 3 3 1 1 1]
  Mux2 : Mux
  Mux3 : Mux  Inputs=[1 1 4 1]
  Terminator_{1..28} (28 alike) : Terminator
  a11 : Fcn  Expr=u[12]*((u[10]+u[7])*cos(u[11])-u[8]*sin(u[11]))-u[3]
  a12 : Fcn  Expr=-u[6]
  a21 : Fcn  Expr=u[12]*u[9]*sin(u[11])-u[2]
  a22 : Fcn  Expr=u[12]*(u[10]+u[7])-u[5]
  alphadot : Fcn  Expr=(u[6]*u[1]-u[4]*u[2])/u[7]
  b1 : Fcn  Expr=u[3]-u[14]*(u[12]-u[5]*(u[13]+u[7])+u[4]*u[8])
  b2 : Fcn  Expr=u[2]-u[14]*(u[11]+u[6]*(u[13]+u[7])-u[4]*u[9])
  betadot : Fcn  Expr=(-u[5]*u[1]+u[3]*u[2])/u[7]
  det : Fcn  Expr=u[1]*u[4]-u[2]*u[3]
  states : Demux  Outputs=12
      settings: DisplayOption=none
  adot : Outport  VectorParamsAs1DForOutWhenUnconnected=off
  bdot : Outport  Port=2  VectorParamsAs1DForOutWhenUnconnected=off
  wires:
  states/12 -> Terminator_28/1
  states/11 -> Terminator_27/1
  states/10 -> Terminator_26/1
  states/9 -> Terminator_25/1
  states/8 -> Terminator_24/1
  states/7 -> Terminator_23/1
  states/5 -> Terminator_22/1
  states/3 -> Terminator_21/1
  states/2 -> Terminator_20/1
  states/1 -> Terminator_19/1
  Demux5/4 -> Terminator_18/1
  Demux5/3 -> Terminator_17/1
  Demux5/2 -> Terminator_16/1
  Demux4/4 -> Terminator_15/1
  Demux4/3 -> Terminator_14/1
  Demux4/2 -> Terminator_13/1
  Demux3/4 -> Terminator_12/1
  Demux3/3 -> Terminator_11/1
  Demux3/2 -> Terminator_10/1
  Demux2/4 -> Terminator_9/1
  Demux2/3 -> Terminator_8/1
  Demux2/2 -> Terminator_7/1
  Demux1/4 -> Terminator_6/1
  Demux1/3 -> Terminator_5/1
  Demux1/2 -> Terminator_4/1
  Demux/4 -> Terminator_3/1
  Demux/3 -> Terminator_2/1
  Demux/2 -> Terminator_1/1
  states/4 -> Mux/5, Mux1/4
  Demux2/1 -> Mux/3, Mux1/3
  Demux3/1 -> Mux/4
  winddot/1 -> Demux3/1
  states/6 -> Mux1/5
  Mux3/1 -> betadot/1, alphadot/1
  Mux/1 -> b2/1, b1/1
  b1/1 -> Mux3/1
  b2/1 -> Mux3/2
  det/1 -> Mux3/4
  Mux2/1 -> det/1, Mux3/3
  a22/1 -> Mux2/4
  a21/1 -> Mux2/3
  a12/1 -> Mux2/2
  a11/1 -> Mux2/1
  x/1 -> states/1
  Demux5/1 -> Mux1/2
  alphadot/1 -> adot/1
  betadot/1 -> bdot/1
  ypqr/1 -> Demux1/1
  Demux1/1 -> Mux/2
  Demux/1 -> Mux/1
  Ftot/1 -> Demux/1
  Demux4/1 -> Mux1/1
  Fbdot/1 -> Demux5/1
  Fadot/1 -> Demux4/1
  wind/1 -> Demux2/1
  mass/1 -> Mux1/6, Mux/6
  Mux1/1 -> a21/1, a22/1, a11/1, a12/1

== system c_citation/Cessna Citation 500/Citation model DASMAT/AIRCRAFT MODEL/LANDING GEAR/Landing Gear model/Left Main Gear/Axes Transformation Heading attached vertical axis to body axis ==
  Fmu FS FV phi theta : Inport
  FX : Fcn  Expr=-cos(u[5])*u[1]+0*u[2]+sin(u[5])*u[3]
  FY : Fcn  Expr=-sin(u[5])*sin(u[4])*u[1]-cos(u[4])*u[2]-cos(u[5])*sin(u[4])*u[3]
  FZ : Fcn  Expr=-sin(u[5])*cos(u[4])*u[1]+sin(u[4])*u[2]-cos(u[5])*cos(u[4])*u[3]
  Mux1 : Mux  Inputs=3
  FX FY FZ : Outport  VectorParamsAs1DForOutWhenUnconnected=off
  wires:
  Fmu FS FV phi theta/1 -> FX/1, FY/1, FZ/1
  FX/1 -> Mux1/1
  FY/1 -> Mux1/2
  FZ/1 -> Mux1/3
  Mux1/1 -> FX FY FZ/1

== system c_citation/Cessna Citation 500/Citation model DASMAT/AIRCRAFT MODEL/LANDING GEAR/Landing Gear model/Left Main Gear/Calculation of the Moments ==
  FX FY FZ : Inport
  L : Fcn  Expr=0*u[1]-zl1*u[2]+yl1*u[3]
  M : Fcn  Expr=zl1*u[1]+0*u[2]-xl1*u[3]
  Mux2 : Mux  Inputs=3
  N : Fcn  Expr=-yl1*u[1]+xl1*u[2]+0*u[3]
  L M N : Outport  VectorParamsAs1DForOutWhenUnconnected=off
  wires:
  L/1 -> Mux2/1
  M/1 -> Mux2/2
  N/1 -> Mux2/3
  FX FY FZ/1 -> M/1, L/1, N/1
  Mux2/1 -> L M N/1

== system c_citation/Cessna Citation 500/Citation model DASMAT/AIRCRAFT MODEL/LANDING GEAR/Landing Gear model/Left Main Gear/FV Vertical Force ==
  In1 : Inport
  B : Fcn  Expr=(u[2]/kt1)-u[1]-deltagmax1
  C : Fcn  Expr=(deltagmax1/kt1)*(P1+u[2]-(kt1*u[1]))
  FD damping force : Fcn  Expr=cv1*u[1]
  FV : Fcn  Expr=kt1*(u[1]-u[2])
  FV No ground contact : Constant  Value=0
  Mux1 : Mux  Inputs=2
  Mux2 : Mux  Inputs=2
  Mux3 : Mux  Inputs=2
  No negative Strut deflection : Saturate  UpperLimit=inf  LowerLimit=0
  Prevent Earth from pulling a/c when FD>FV : Saturate  UpperLimit=inf  LowerLimit=0
  Strut deflection : Fcn  Expr=0.5*(-u[1]-sqrt(u[1]*u[1]+4*u[2]))
  Switch1 : Switch  SaturateOnIntegerOverflow=on  InputSameDT=on
  deltag : Fcn  Expr=zl1-u[10]-xl1*sin(u[8])+yl1*sin(u[7])
  deltagdot : Fcn  Expr=-u[13]-xl1*u[2]*cos(u[8])+yl1*u[1]*cos(u[7])
  Out1 : Outport  VectorParamsAs1DForOutWhenUnconnected=off
  wires:
  In1/1 -> deltag/1, deltagdot/1
  deltagdot/1 -> FD damping force/1
  Strut deflection/1 -> No negative Strut deflection/1
  FD damping force/1 -> Mux1/2
  Mux1/1 -> B/1, C/1
  B/1 -> Mux2/1
  C/1 -> Mux2/2
  Mux2/1 -> Strut deflection/1
  Mux3/1 -> FV/1
  No negative Strut deflection/1 -> Mux3/2
  deltag/1 -> Mux1/1, Mux3/1, Switch1/2
  FV/1 -> Prevent Earth from pulling a/c when FD>FV/1
  FV No ground contact/1 -> Switch1/3
  Prevent Earth from pulling a/c when FD>FV/1 -> Switch1/1
  Switch1/1 -> Out1/1

== system c_citation/Cessna Citation 500/Citation model DASMAT/AIRCRAFT MODEL/LANDING GEAR/Landing Gear model/Nose Gear/Axes Transformation Heading attached vertical axis to body axis ==
  Fmu FS FV phi theta : Inport
  FX : Fcn  Expr=-cos(u[5])*u[1]+0*u[2]+sin(u[5])*u[3]
  FY : Fcn  Expr=-sin(u[5])*sin(u[4])*u[1]-cos(u[4])*u[2]-cos(u[5])*sin(u[4])*u[3]
  FZ : Fcn  Expr=-sin(u[5])*cos(u[4])*u[1]+sin(u[4])*u[2]-cos(u[5])*cos(u[4])*u[3]
  Mux1 : Mux  Inputs=3
  FX FY FZ : Outport  VectorParamsAs1DForOutWhenUnconnected=off
  wires:
  Fmu FS FV phi theta/1 -> FX/1, FY/1, FZ/1
  FX/1 -> Mux1/1
  FY/1 -> Mux1/2
  FZ/1 -> Mux1/3
  Mux1/1 -> FX FY FZ/1

== system c_citation/Cessna Citation 500/Citation model DASMAT/AIRCRAFT MODEL/LANDING GEAR/Landing Gear model/Nose Gear/Calculation of the Moments ==
  FX FY FZ : Inport
  L : Fcn  Expr=0*u[1]-zl3*u[2]+yl3*u[3]
  M : Fcn  Expr=zl3*u[1]+0*u[2]-xl3*u[3]
  Mux2 : Mux  Inputs=3
  N : Fcn  Expr=-yl3*u[1]+xl3*u[2]+0*u[3]
  L M N : Outport  VectorParamsAs1DForOutWhenUnconnected=off
  wires:
  L/1 -> Mux2/1
  M/1 -> Mux2/2
  N/1 -> Mux2/3
  FX FY FZ/1 -> M/1, L/1, N/1
  Mux2/1 -> L M N/1

== system c_citation/Cessna Citation 500/Citation model DASMAT/AIRCRAFT MODEL/LANDING GEAR/Landing Gear model/Nose Gear/F Vertical Force ==
  In1 : Inport
  B : Fcn  Expr=(u[2]/kt3)-u[1]-deltagmax3
  C : Fcn  Expr=(deltagmax3/kt3)*(P3+u[2]-(kt3*u[1]))
  FD damping force : Fcn  Expr=cv3*u[1]
  FV : Fcn  Expr=kt3*(u[1]-u[2])
  FV No ground contact : Constant  Value=0
  Mux1 : Mux  Inputs=2
  Mux2 : Mux  Inputs=2
  Mux3 : Mux  Inputs=2
  No negative Strut deflection : Saturate  UpperLimit=inf  LowerLimit=0
  Prevent Earth from pulling a/c when FD>FV : Saturate  UpperLimit=inf  LowerLimit=0
  Strut deflection : Fcn  Expr=0.5*(-u[1]-sqrt(u[1]*u[1]+4*u[2]))
  Switch1 : Switch  SaturateOnIntegerOverflow=on  InputSameDT=on
  deltag : Fcn  Expr=zl3-u[10]-xl3*sin(u[8])+yl3*sin(u[7])
  deltagdot : Fcn  Expr=-u[13]-xl3*u[2]*cos(u[8])+yl3*u[1]*cos(u[7])
  Out1 : Outport  VectorParamsAs1DForOutWhenUnconnected=off
  wires:
  In1/1 -> deltag/1, deltagdot/1
  deltagdot/1 -> FD damping force/1
  Strut deflection/1 -> No negative Strut deflection/1
  FD damping force/1 -> Mux1/2
  Mux1/1 -> B/1, C/1
  B/1 -> Mux2/1
  C/1 -> Mux2/2
  Mux2/1 -> Strut deflection/1
  Mux3/1 -> FV/1
  No negative Strut deflection/1 -> Mux3/2
  deltag/1 -> Mux1/1, Mux3/1, Switch1/2
  FV/1 -> Prevent Earth from pulling a/c when FD>FV/1
  FV No ground contact/1 -> Switch1/3
  Prevent Earth from pulling a/c when FD>FV/1 -> Switch1/1
  Switch1/1 -> Out1/1

== system c_citation/Cessna Citation 500/Citation model DASMAT/AIRCRAFT MODEL/LANDING GEAR/Landing Gear model/Right Main Gear/Axes Transformation Heading attached vertical axis to body axis ==
  Fmu FS FV phi theta : Inport
  FX : Fcn  Expr=-cos(u[5])*u[1]+0*u[2]+sin(u[5])*u[3]
  FY : Fcn  Expr=-sin(u[5])*sin(u[4])*u[1]-cos(u[4])*u[2]-cos(u[5])*sin(u[4])*u[3]
  FZ : Fcn  Expr=-sin(u[5])*cos(u[4])*u[1]+sin(u[4])*u[2]-cos(u[5])*cos(u[4])*u[3]
  Mux1 : Mux  Inputs=3
  FX FY FZ : Outport  VectorParamsAs1DForOutWhenUnconnected=off
  wires:
  Fmu FS FV phi theta/1 -> FX/1, FY/1, FZ/1
  FX/1 -> Mux1/1
  FY/1 -> Mux1/2
  FZ/1 -> Mux1/3
  Mux1/1 -> FX FY FZ/1

== system c_citation/Cessna Citation 500/Citation model DASMAT/AIRCRAFT MODEL/LANDING GEAR/Landing Gear model/Right Main Gear/Calculation of the Moments ==
  FX FY FZ : Inport
  L : Fcn  Expr=0*u[1]-zl2*u[2]+yl2*u[3]
  M : Fcn  Expr=zl2*u[1]+0*u[2]-xl2*u[3]
  Mux2 : Mux  Inputs=3
  N : Fcn  Expr=-yl2*u[1]+xl2*u[2]+0*u[3]
  L M N : Outport  VectorParamsAs1DForOutWhenUnconnected=off
  wires:
  L/1 -> Mux2/1
  M/1 -> Mux2/2
  N/1 -> Mux2/3
  FX FY FZ/1 -> M/1, L/1, N/1
  Mux2/1 -> L M N/1

== system c_citation/Cessna Citation 500/Citation model DASMAT/AIRCRAFT MODEL/LANDING GEAR/Landing Gear model/Right Main Gear/FV Vertical Force ==
  In1 : Inport
  B : Fcn  Expr=(u[2]/kt2)-u[1]-deltagmax2
  C : Fcn  Expr=(deltagmax2/kt2)*(P2+u[2]-(kt2*u[1]))
  FD damping force : Fcn  Expr=cv2*u[1]
  FV : Fcn  Expr=kt2*(u[1]-u[2])
  FV No ground contact : Constant  Value=0
  Mux1 : Mux  Inputs=2
  Mux2 : Mux  Inputs=2
  Mux3 : Mux  Inputs=2
  No negative Strut deflection : Saturate  UpperLimit=inf  LowerLimit=0
  Prevent Earth from pulling a/c when FD>FV : Saturate  UpperLimit=inf  LowerLimit=0
  Strut deflection : Fcn  Expr=0.5*(-u[1]-sqrt(u[1]*u[1]+4*u[2]))
  Switch1 : Switch  SaturateOnIntegerOverflow=on  InputSameDT=on
  deltag : Fcn  Expr=zl2-u[10]-xl2*sin(u[8])+yl2*sin(u[7])
  deltagdot : Fcn  Expr=-u[13]-xl2*u[2]*cos(u[8])+yl2*u[1]*cos(u[7])
  Out1 : Outport  VectorParamsAs1DForOutWhenUnconnected=off
  wires:
  In1/1 -> deltag/1, deltagdot/1
  deltagdot/1 -> FD damping force/1
  Strut deflection/1 -> No negative Strut deflection/1
  FD damping force/1 -> Mux1/2
  Mux1/1 -> B/1, C/1
  B/1 -> Mux2/1
  C/1 -> Mux2/2
  Mux2/1 -> Strut deflection/1
  Mux3/1 -> FV/1
  No negative Strut deflection/1 -> Mux3/2
  deltag/1 -> Mux1/1, Mux3/1, Switch1/2
  FV/1 -> Prevent Earth from pulling a/c when FD>FV/1
  FV No ground contact/1 -> Switch1/3
  Prevent Earth from pulling a/c when FD>FV/1 -> Switch1/1
  Switch1/1 -> Out1/1

== system c_citation/Cessna Citation 500/Citation model DASMAT/AIRCRAFT MODEL/LANDING GEAR/Landing Gear model/Tail Scraper/Axes Transformation Heading attached vertical axis to body axis ==
  Fmu FS FV phi theta : Inport
  FX : Fcn  Expr=-cos(u[5])*u[1]+0*u[2]+sin(u[5])*u[3]
  FY : Fcn  Expr=-sin(u[5])*sin(u[4])*u[1]-cos(u[4])*u[2]-cos(u[5])*sin(u[4])*u[3]
  FZ : Fcn  Expr=-sin(u[5])*cos(u[4])*u[1]+sin(u[4])*u[2]-cos(u[5])*cos(u[4])*u[3]
  Mux1 : Mux  Inputs=3
  FX FY FZ : Outport  VectorParamsAs1DForOutWhenUnconnected=off
  wires:
  Fmu FS FV phi theta/1 -> FX/1, FY/1, FZ/1
  FX/1 -> Mux1/1
  FY/1 -> Mux1/2
  FZ/1 -> Mux1/3
  Mux1/1 -> FX FY FZ/1

== system c_citation/Cessna Citation 500/Citation model DASMAT/AIRCRAFT MODEL/LANDING GEAR/Landing Gear model/Tail Scraper/Calculation of the Moments ==
  FX FY FZ : Inport
  L : Fcn  Expr=0*u[1]-zl4*u[2]+yl4*u[3]
  M : Fcn  Expr=zl4*u[1]+0*u[2]-xl4*u[3]
  Mux2 : Mux  Inputs=3
  N : Fcn  Expr=-yl4*u[1]+xl4*u[2]+0*u[3]
  L M N : Outport  VectorParamsAs1DForOutWhenUnconnected=off
  wires:
  L/1 -> Mux2/1
  M/1 -> Mux2/2
  N/1 -> Mux2/3
  FX FY FZ/1 -> M/1, L/1, N/1
  Mux2/1 -> L M N/1

== system c_citation/Cessna Citation 500/Citation model DASMAT/AIRCRAFT MODEL/LANDING GEAR/Landing Gear model/Tail Scraper/FV Vertical Force ==
  In1 : Inport
  FD damping force : Fcn  Expr=cv4*u[1]
  FV : Fcn  Expr=P4*u[1]+u[2]
  FV No ground contact : Constant  Value=0
  Max Strut Deflection : Saturate  UpperLimit=deltagmax4  LowerLimit=-inf
  Mux1 : Mux  Inputs=2
  Prevent Earth from pulling a/c when FD>FV : Saturate  UpperLimit=inf  LowerLimit=0
  Scope6 : Scope
  Switch : Switch  SaturateOnIntegerOverflow=on  InputSameDT=on
  deltag : Fcn  Expr=zl4-u[10]-xl4*sin(u[8])+yl4*sin(u[7])
  deltagdot : Fcn  Expr=-u[13]-xl4*u[2]*cos(u[8])+yl4*u[1]*cos(u[7])
  Out1 : Outport  VectorParamsAs1DForOutWhenUnconnected=off
  wires:
  In1/1 -> deltag/1, deltagdot/1
  deltagdot/1 -> FD damping force/1
  deltag/1 -> Max Strut Deflection/1
  Max Strut Deflection/1 -> Scope6/1, Mux1/1, Switch/2
  Mux1/1 -> FV/1
  FD damping force/1 -> Mux1/2
  FV/1 -> Prevent Earth from pulling a/c when FD>FV/1
  Prevent Earth from pulling a/c when FD>FV/1 -> Switch/1
  FV No ground contact/1 -> Switch/3
  Switch/1 -> Out1/1

== system c_citation/Cessna Citation 500/Citation model DASMAT/AIRCRAFT MODEL/WIND//TURBULENCE/Logarithmic Wind model/Logarithmic Wind model/Vwind915 ==
  Constant : Constant  Value=0
  Parameter : Integrator  InitialCondition=Vw915
  Out1 : Outport  VectorParamsAs1DForOutWhenUnconnected=off
  wires:
  Constant/1 -> Parameter/1
  Parameter/1 -> Out1/1

== system c_citation/Cessna Citation 500/Citation model DASMAT/AIRCRAFT MODEL/WIND//TURBULENCE/Logarithmic Wind model/Logarithmic Wind model/Windddirection ==
  Constant : Constant  Value=0
  Parameter : Integrator  InitialCondition=winddir
  Out1 : Outport  VectorParamsAs1DForOutWhenUnconnected=off
  wires:
  Constant/1 -> Parameter/1
  Parameter/1 -> Out1/1

== system c_citation/Cessna Citation 500/Citation model DASMAT/AIRCRAFT MODEL/AFM/Aeromod/SubSystem/model/CDCAL ==
  in_1 : Inport
  Abs : Abs  SaturateOnIntegerOverflow=on
  Abs1 : Abs  SaturateOnIntegerOverflow=on
  CD : Sum  Inputs=++++++++  InputSameDT=on  SaturateOnIntegerOverflow=on  OutDataTypeStr=Inherit: Same as first input
  CDAF : Lookup2D  RowIndex=matdaf(2:23,1)  ColumnIndex=matdaf(1,2:23)  Table=matdaf(2:23,2:23)  SaturateOnIntegerOverflow=on  InputSameDT=on
  CDAM : Lookup2D  RowIndex=matdam(2:23,1)  ColumnIndex=matdam(1,2:23)  Table=matdam(2:23,2:23)  SaturateOnIntegerOverflow=on  InputSameDT=on
  CDBAS : Sum  InputSameDT=on  SaturateOnIntegerOverflow=on  OutDataTypeStr=Inherit: Same as first input
  CDBBF : Lookup2D  RowIndex=matdbbf(2:18,1)  ColumnIndex=matdbbf(1,2:18)  Table=matdbbf(2:18,2:18)  SaturateOnIntegerOverflow=on  InputSameDT=on
  CDDE : Product  InputSameDT=on  SaturateOnIntegerOverflow=on  OutDataTypeStr=Inherit: Same as first input
  CDEAF : Lookup2D  RowIndex=matdeaf(2:23,1)  ColumnIndex=matdeaf(1,2:23)  Table=matdeaf(2:23,2:23)  SaturateOnIntegerOverflow=on  InputSameDT=on
  CDGAF : Lookup2D  RowIndex=matdgaf(2:4,1)  ColumnIndex=matdgaf(1,2:4)  Table=matdgaf(2:4,2:4)  SaturateOnIntegerOverflow=on  InputSameDT=on
  CDGE : Product  InputSameDT=on  SaturateOnIntegerOverflow=on  OutDataTypeStr=Inherit: Same as first input
  CDQ : Product  InputSameDT=on  SaturateOnIntegerOverflow=on  OutDataTypeStr=Inherit: Same as first input
  CDQAF : Lookup2D  RowIndex=matdqaf(2:23,1)  ColumnIndex=matdqaf(1,2:23)  Table=matdqaf(2:23,2:23)  SaturateOnIntegerOverflow=on  InputSameDT=on
  CDR : Product  Inputs=3  InputSameDT=on  SaturateOnIntegerOverflow=on  OutDataTypeStr=Inherit: Same as first input
  CDRUAF : Lookup2D  RowIndex=matruaf(2:3,1)  ColumnIndex=matruaf(1,2:3)  Table=matruaf(2:3,2:3)  SaturateOnIntegerOverflow=on  InputSameDT=on
  CDUAF : Lookup2D  RowIndex=matduaf(2:23,1)  ColumnIndex=matduaf(1,2:23)  Table=matduaf(2:23,2:23)  SaturateOnIntegerOverflow=on  InputSameDT=on
  CDUC : Product  InputSameDT=on  SaturateOnIntegerOverflow=on  OutDataTypeStr=Inherit: Same as first input
  CDWAW : Lookup2D  RowIndex=matdwaw(2:7,1)  ColumnIndex=matdwaw(1,2:7)  Table=matdwaw(2:7,2:7)  SaturateOnIntegerOverflow=on  InputSameDT=on
  Demux : Demux  Outputs=[1 1 1 1 1 1 1 1 1 1 1 1 1 1 1 1 1 1]
      settings: DisplayOption=none
  KBASD : Subsystem
  KGEDHR : Lookup  InputValues=matedhr(1,:)  Table=matedhr(2,:)  SaturateOnIntegerOverflow=on
  KUUT : Lookup  InputValues=matuut(1,:)  Table=matuut(2,:)  SaturateOnIntegerOverflow=on
  Prod : Product  InputSameDT=on  SaturateOnIntegerOverflow=on  OutDataTypeStr=Inherit: Same as first input
  Terminator_{1..7} (7 alike) : Terminator
  out_1 : Outport  VectorParamsAs1DForOutWhenUnconnected=off
  wires:
  Demux/16 -> Terminator_7/1
  Demux/13 -> Terminator_6/1
  Demux/12 -> Terminator_5/1
  Demux/11 -> Terminator_4/1
  Demux/6 -> Terminator_3/1
  Demux/3 -> Terminator_2/1
  Demux/1 -> Terminator_1/1
  Demux/7 -> KBASD/1(hcg), KGEDHR/1
  Demux/18 -> KBASD/3(VEAS)
  Demux/2 -> CDQ/1
  Demux/5 -> Abs1/1
  Demux/8 -> CDDE/1
  Demux/9 -> Abs/1
  Demux/15 -> KUUT/1
  Demux/17 -> CDAM/1
  KUUT/1 -> CDUC/2
  CDGAF/1 -> CDGE/1
  CDR/1 -> CD/6
  CDQ/1 -> CD/5
  CDWAW/1 -> CD/3
  CDDE/1 -> CD/2
  CDRUAF/1 -> CDR/3
  CDQAF/1 -> CDQ/2
  CDEAF/1 -> CDDE/2
  Abs/1 -> CDWAW/1
  Abs1/1 -> CDBBF/2
  CD/1 -> out_1/1
  Demux/10 -> CDR/1, CDR/2
  Demux/14 -> CDAF/1, CDRUAF/1, CDUAF/1, CDGAF/1, CDQAF/1, CDBBF/1, CDEAF/1, KBASD/2(deltaf)
  KGEDHR/1 -> CDGE/2
  Demux/4 -> CDRUAF/2, CDUAF/2, CDGAF/2, CDQAF/2, CDWAW/2, CDEAF/2, CDAF/2, CDAM/2
  CDAF/1 -> Prod/1
  KBASD/1(KBASD) -> Prod/2
  CDUAF/1 -> CDUC/1
  CDUC/1 -> CD/7
  CDGE/1 -> CD/8
  CDBBF/1 -> CD/4
  Prod/1 -> CDBAS/2
  CDAM/1 -> CDBAS/1
  CDBAS/1 -> CD/1
  in_1/1 -> Demux/1
